simulink model "message_carrier"  (R2019b)
settings: Solver=VariableStepAuto  StartTime=0.0  StopTime=2  RelTol=1e-3
libraries: powerlib x1
settings Model: Creator=Lenovo  LastModifiedBy=Lenovo

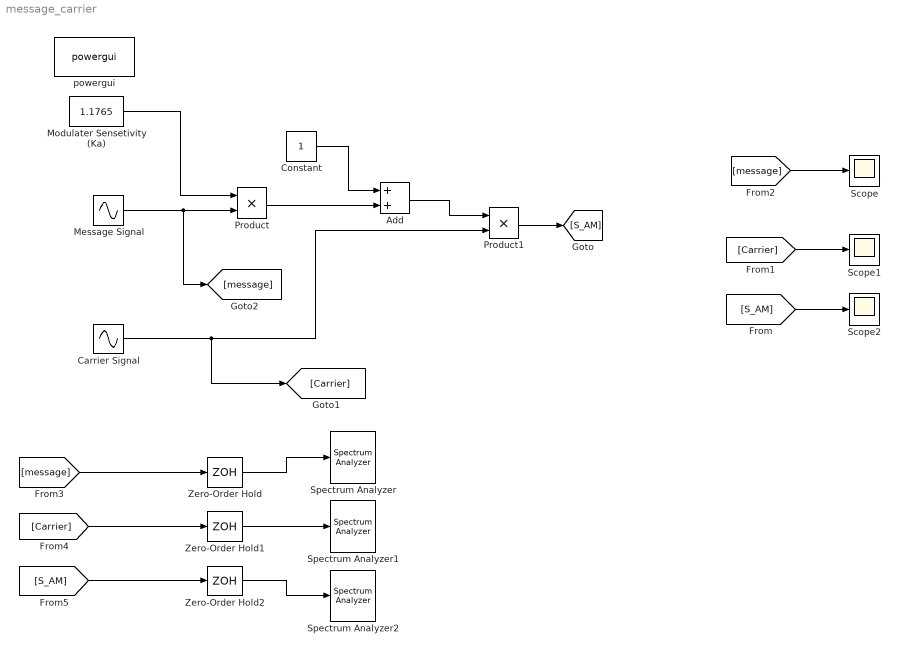
== system message_carrier ==
  Add : Sum
  Carrier Signal : Sin  Frequency=2*pi*15000  SampleTime=0
  Constant : Constant
  Message Signal : Sin  Amplitude=0.85  Frequency=2*pi*1000  SampleTime=0
  Modulater Sensetivity (Ka) : Constant  Value=1.1765
  Product : Product
  Product1 : Product
  Scope : Scope
  Scope1 : Scope
  Scope2 : Scope
  Spectrum Analyzer : SpectrumAnalyzer
  Spectrum Analyzer1 : SpectrumAnalyzer
  Spectrum Analyzer2 : SpectrumAnalyzer
  Zero-Order Hold : ZeroOrderHold  SampleTime=1/(10*1e3)
  Zero-Order Hold1 : ZeroOrderHold  SampleTime=1/(10*15e3)
  Zero-Order Hold2 : ZeroOrderHold  SampleTime=1/(10*15e3)
  powergui : powerlib/powergui  Priority=1  SimulationMode=Continuous  SampleTime=50e-6  frequency=60  Iterations=50  frequencyindice=60  Pbase=100e6  ErrMax=1e-4  UnitsV=kV  UnitsW=MW  buscounter=0  FunctionMessages=off  echomessages=off  EnableUseOfTLC=off  CurrentSourceSwitches=off  DisableSnubberDevices=off  DisableRonSwitches=off  DisableVfSwitches=off  DisplayEquations=off  AutomaticDiscreteSolvers=off  SolverType=Tustin/Backward Euler (TBE)  Interpol=off  ExternalGateDelay=off  methode=off  Ts=100  x0status=blocks  SPID=on  SwTol=0  HookPort=off  NonlinearTolerance=1e-4  nMaxIteration=100  ContinueOnMaxIteration=off  RestoreLinks=warning  ResistiveCurrentMeasurement=off  Frange=[0:2:500]  Ylog=off  Xlog=on  ShowGrid=off  save=off  variable=ZData  structure=0  ZoomFFT=off  StartTime=0.0  cycles=1  DisplayStyle=1  fundamental=60  FreqAxis=off  MaxFrequency=1000  frequencyindicesteady=1  RmsSteady=1  display=off
      settings: SourceProductName=Simscape Electrical
  wires:
  Modulater Sensetivity (Ka)/1 -> Product/1
  [message] -> Scope/1
  [message] -> Zero-Order Hold/1
  [S_AM] -> Scope2/1
  Message Signal/1 -> [message], Product/2
  Zero-Order Hold1/1 -> Spectrum Analyzer1/1
  [Carrier] -> Zero-Order Hold1/1
  [S_AM] -> Zero-Order Hold2/1
  [Carrier] -> Scope1/1
  Zero-Order Hold/1 -> Spectrum Analyzer/1
  Product1/1 -> [S_AM]
  Product/1 -> Add/2
  Zero-Order Hold2/1 -> Spectrum Analyzer2/1
  Add/1 -> Product1/1
  Constant/1 -> Add/1
  Carrier Signal/1 -> [Carrier], Product1/2
